simulink model "adcs_v16_integral_light_sun_sgp_igrf"  (Simulink 7.4)
settings: Solver=ode4  StartTime=0.0  StopTime=5000  FixedStep=s_SIM_STEP_SIZE  RelTol=1e-3
values from neighbouring files (symbols this model uses):
  A = ((T_SIDE + .29)*1e-3)^2    [constants_v13.m]    (also in constants_v15.m; constants_v15_Pow.m; constants_v15_Pow_ss_error.m; constants_v16_integral_kartavya.m)
  Bstar = SGP4dragp    (= -3.5889e-05)    [constants_v16_integral_light_sun_sgp_igrf_power_13Dec2011.m]    (also in getOrbitData.m = SGP4dragp; sgp.m = modTLE(4))
  Ca_Solar_Drag = 1.4    [constants_v13.m]    (also in constants_v15.m; constants_v15_Pow.m; constants_v15_Pow_ss_error.m; constants_v16_integral_kartavya.m)
  Cd = 2.2    [constants_v13.m]    (also in constants_v15.m; constants_v15_Pow.m; constants_v15_Pow_ss_error.m; constants_v16_integral_kartavya.m)
  check_time = 60000    [constants_v13.m]    (also in constants_v15.m = 10000; constants_v15_Pow.m = 10000; constants_v15_Pow_ss_error.m = 10000; constants_v16_integral_kartavya.m = 10000)
  ddn0 = 6*2*pi*SGPdragp2/(1440^3)    (= 0)    [constants_v16_integral_light_sun_sgp_igrf_power_13Dec2011.m]    (also in getOrbitData.m = 6*2*pi*SGPdragp2/(1440^3); sgp.m = modTLE(3))
  dn0 = 2*2*pi*SGPdragp1/(1440^2)    (= -4.7632944169e-11)    [constants_v16_integral_light_sun_sgp_igrf_power_13Dec2011.m]    (also in getOrbitData.m = 2*2*pi*SGPdragp1/(1440^2); sgp.m = modTLE(2))
  equinox = datenum('21-Mar-2010 12:0:0')    [constants_v13.m]    (also in constants_v15.m; constants_v15_Pow.m; constants_v15_Pow_ss_error.m; constants_v16_integral_kartavya.m)
  err_SGP = 0    [constants_v16_integral_kartavya.m]    (also in constants_v16_integral_light_sun_sgp_igrf_power_13Dec2011.m)
  i0 = pi*orbInc/180    (= 1.72229090587)    [constants_v16_integral_light_sun_sgp_igrf_power_13Dec2011.m]    (also in getOrbitData.m = pi*orbInc/180; sgp.m = modTLE(5))
  I_MAX = 0.5    [constants_v13.m]    (also in constants_v15.m; constants_v15_Pow.m; constants_v15_Pow_ss_error.m; constants_v16_integral_kartavya.m)
  I_TORQUER = 3.6 / 7.31    (= 0.492476060192)    [constants_v13.m]    (also in constants_v15.m; constants_v15_Pow.m; constants_v15_Pow_ss_error.m; constants_v16_integral_kartavya.m)
  Kd = 2* m_INERTIA / (s_numOrbits * T_ORBIT )    [constants_v13.m]    (also in constants_v15.m = m_INERTIA * (2 + delta)* zeta * w; constants_v15_Pow.m = m_INERTIA * (2 + delta)* zeta * w; constants_v15_Pow_ss_error.m = m_INERTIA * (2 + delta)* zeta * w; constants_v16_integral_kartavya.m = m_INERTIA * (2 + delta)* zeta * w)
  Kdetumb = K_det*eye(3)    [constants_v13.m]    (also in constants_v15.m; constants_v15_Pow.m; constants_v15_Pow_ss_error.m; constants_v16_integral_kartavya.m)
  Ki = m_INERTIA * delta * zeta * w^3    [constants_v15.m]    (also in constants_v15_Pow.m; constants_v15_Pow_ss_error.m; constants_v16_integral_kartavya.m; constants_v16_integral_light_sun_sgp_igrf_power_13Dec2011.m)
  Kp = m_INERTIA / (s_numOrbits * T_ORBIT * zeta)^2    [constants_v13.m]    (also in constants_v15.m = m_INERTIA * (w*w + 2*delta*zeta^2*w^2); constants_v15_Pow.m = m_INERTIA * (w*w + 2*delta*zeta^2*w^2); constants_v15_Pow_ss_error.m = m_INERTIA * (w*w + 2*delta*zeta^2*w^2); constants_v16_integral_kartavya.m = m_INERTIA * (w*w + 2*delta*zeta^2*w^2))
  M0 = pi*meanAno/180    (= 0)    [constants_v16_integral_light_sun_sgp_igrf_power_13Dec2011.m]    (also in getOrbitData.m = pi*meanAno/180; sgp.m = modTLE(9))
  m_INERTIA = [Ixx Ixy Ixz; Ixy Iyy Iyz; Ixz Iyz Izz]    [constants_v13.m]    (also in constants_v15.m; constants_v15_Pow.m = 1*[Ixx Ixy Ixz; Ixy Iyy Iyz; Ixz Iyz Izz]; constants_v15_Pow_ss_error.m = 1*[Ixx Ixy Ixz; Ixy Iyy Iyz; Ixz Iyz Izz]; constants_v16_integral_kartavya.m)
  mu = 6.673e-11*5.9742e24    (= 398658366000000)    [constants_v13.m]    (also in constants_v15.m; constants_v15_Pow.m; constants_v15_Pow_ss_error.m; constants_v16_integral_kartavya.m)
  N = 40    [constants_v13.m]    (also in constants_v15.m; constants_v15_Pow.m; constants_v15_Pow_ss_error.m; constants_v16_integral_kartavya.m)
  n0 = 2*pi*meanMo/1440    [constants_v16_integral_light_sun_sgp_igrf_power_13Dec2011.m]    (also in getOrbitData.m; sgp.m = modTLE(10))
  Ohm0 = pi*rghtAsc/180    (= 3.21433797681)    [constants_v16_integral_light_sun_sgp_igrf_power_13Dec2011.m]    (also in getOrbitData.m = pi*rghtAsc/180; sgp.m = modTLE(6))
  P_momentum_flux_from_the_sun = 4.4e-6    (= 4.4e-06)    [constants_v13.m]    (also in constants_v15.m; constants_v15_Pow.m; constants_v15_Pow_ss_error.m; constants_v16_integral_kartavya.m)
  q_BI0 = euler2qBI(roll0,pitch0,yaw0)    [constants_v13.m]    (also in constants_v15.m; constants_v15_Pow.m; constants_v15_Pow_ss_error.m; constants_v16_integral_kartavya.m)
  revNo = 1    [constants_v16_integral_kartavya.m]    (also in constants_v16_integral_light_sun_sgp_igrf_power_13Dec2011.m; precalcs.m; sgp.m = modTLE(11))
  s_AU = 159597870610    [constants_v16_integral_kartavya.m]    (also in constants_v16_integral_light_sun_sgp_igrf_power_13Dec2011.m; light_calc.m)
  s_FRAME_SIZE = 2    [constants_v13.m]    (also in constants_v15.m; constants_v15_Pow.m; constants_v15_Pow_ss_error.m; constants_v16_integral_kartavya.m)
  s_m_MAX = 0.95    [constants_v13.m]    (also in constants_v15.m; constants_v15_Pow.m; constants_v15_Pow_ss_error.m; constants_v16_integral_kartavya.m)
  s_MAG_B = 2.5e-5    (= 2.5e-05)    [constants_v13.m]    (also in constants_v15.m; constants_v15_Pow.m; constants_v15_Pow_ss_error.m; constants_v16_integral_kartavya.m)
  s_MAGMETER_WEIGHT = .9    (= 0.9)    [constants_v13.m]    (also in constants_v15.m; constants_v15_Pow.m; constants_v15_Pow_ss_error.m; constants_v16_integral_kartavya.m)
  s_Rearth = 6378164    [constants_v16_integral_kartavya.m]    (also in constants_v16_integral_light_sun_sgp_igrf_power_13Dec2011.m; light_calc.m)
  s_Rsun = 695500000    [constants_v16_integral_kartavya.m]    (also in constants_v16_integral_light_sun_sgp_igrf_power_13Dec2011.m; light_calc.m)
  s_SIM_STEP_SIZE = 0.1    [constants_v13.m]    (also in constants_v15.m; constants_v15_Pow.m; constants_v15_Pow_ss_error.m; constants_v16_integral_kartavya.m)
  s_SS_ADC_gain = 5    [constants_v13.m]    (also in constants_v15.m; constants_v15_Pow.m; constants_v15_Pow_ss_error.m; constants_v16_integral_kartavya.m)
  s_SS_ADC_res = 2^12 - 1    (= 4095)    [constants_v13.m]    (also in constants_v15.m; constants_v15_Pow.m; constants_v15_Pow_ss_error.m; constants_v16_integral_kartavya.m)
  s_SS_MAX_ANGLE = 85    [constants_v13.m]    (also in constants_v15.m; constants_v15_Pow.m; constants_v15_Pow_ss_error.m; constants_v16_integral_kartavya.m)
  s_TAU_W = 60    [constants_v13.m]    (also in constants_v15.m; constants_v15_Pow.m; constants_v15_Pow_ss_error.m; constants_v16_integral_kartavya.m)
  s_x_MAGMETER_BIAS = 50e-9    (= 5e-08)    [constants_v13.m]    (also in constants_v15.m; constants_v15_Pow.m; constants_v15_Pow_ss_error.m; constants_v16_integral_kartavya.m)
  s_YEAR = sime(1) + (sime(2)*30 - 30 + sime(3))/365    [constants_v16_integral_kartavya.m]    (also in constants_v16_integral_light_sun_sgp_igrf_power_13Dec2011.m; precalcs.m)
  side = 0.26    [constants_v13.m]    (also in constants_v15.m; constants_v15_Pow.m; constants_v15_Pow_ss_error.m; constants_v16_integral_kartavya.m)
  Snum = 6    [constants_v13.m]    (also in constants_v15.m; constants_v15_Pow.m; constants_v15_Pow_ss_error.m; constants_v16_integral_kartavya.m)
  t0 = (EpYear*meanYearDays + EpJD + EpTime)*1440    [constants_v16_integral_light_sun_sgp_igrf_power_13Dec2011.m]    (also in getOrbitData.m; sgp.m = modTLE(1))
  TLE_epoch = datenum('18-Oct-2010 10:30:0')    [constants_v16_integral_kartavya.m]    (also in constants_v16_integral_light_sun_sgp_igrf_power_13Dec2011.m; precalcs.m)
  today = datenum('18-Oct-2010 10:30:0')    [constants_v13.m]    (also in constants_v15.m; constants_v15_Pow.m; constants_v15_Pow_ss_error.m; constants_v16_integral_kartavya.m)
  tol_q4 = 0.7    [constants_v13.m]    (also in constants_v15.m = 0.85; constants_v15_Pow.m = 0.85; constants_v15_Pow_ss_error.m = 0.85; constants_v16_integral_kartavya.m = 0.85)
  tol_w = 4e-3    (= 0.004)    [constants_v13.m]    (also in constants_v15.m; constants_v15_Pow.m; constants_v15_Pow_ss_error.m; constants_v16_integral_kartavya.m)
  tolw_n2d = 10e-3    (= 0.01)    [constants_v15.m]    (also in constants_v15_Pow.m; constants_v15_Pow_ss_error.m; constants_v16_integral_kartavya.m; constants_v16_integral_light_sun_sgp_igrf_power_13Dec2011.m)
  Ts_display = 6    [constants_v13.m]    (also in constants_v15.m; constants_v15_Pow.m; constants_v15_Pow_ss_error.m; constants_v16_integral_kartavya.m)
  v_COM_to_COP_b = [.2; 1.75; .2]*1e-2    [constants_v13.m]    (also in constants_v15.m; constants_v15_Pow.m; constants_v15_Pow_ss_error.m; constants_v16_integral_kartavya.m)
  v_S1 = [1 0 0]    [constants_v13.m]    (also in constants_v15.m; constants_v15_Pow.m; constants_v15_Pow_ss_error.m; constants_v16_integral_kartavya.m)
  v_S2 = [-1 0 0]    [constants_v13.m]    (also in constants_v15.m; constants_v15_Pow.m; constants_v15_Pow_ss_error.m; constants_v16_integral_kartavya.m)
  v_S3 = [0 1 0]    [constants_v13.m]    (also in constants_v15.m; constants_v15_Pow.m; constants_v15_Pow_ss_error.m; constants_v16_integral_kartavya.m)
  v_S4 = [0 -1 0]    [constants_v13.m]    (also in constants_v15.m; constants_v15_Pow.m; constants_v15_Pow_ss_error.m; constants_v16_integral_kartavya.m)
  v_S5 = [0 0 1]    [constants_v13.m]    (also in constants_v15.m; constants_v15_Pow.m; constants_v15_Pow_ss_error.m; constants_v16_integral_kartavya.m)
  v_S6 = [0 0 -1]    [constants_v13.m]    (also in constants_v15.m; constants_v15_Pow.m; constants_v15_Pow_ss_error.m; constants_v16_integral_kartavya.m)
  v_x_MOUNTING_THETA_ZYX_BODY_TORQUER = [1; 1; 1]* pi/180    [constants_v13.m]    (also in constants_v15.m; constants_v15_Pow.m; constants_v15_Pow_ss_error.m; constants_v16_integral_kartavya.m)
  w0 = pi*argPer/180    (= 0)    [constants_v16_integral_light_sun_sgp_igrf_power_13Dec2011.m]    (also in getOrbitData.m = pi*argPer/180; sgp.m = modTLE(8))
  wx0 = 2*pi/180    (= 0.0349065850399)    [constants_v13.m]    (also in constants_v15.m = 0.00174532925199; constants_v15_Pow.m = 1.74532925199e-05; constants_v15_Pow_ss_error.m = 2.01533262693e-05; constants_v16_integral_kartavya.m = 0.0174532925199)
  wy0 = 1*pi/180    (= 0.0174532925199)    [constants_v13.m]    (also in constants_v15.m = 0.00174532925199; constants_v15_Pow.m = 1.74532925199e-05; constants_v15_Pow_ss_error.m = 2.01533262693e-05; constants_v16_integral_kartavya.m = 0)
  wz0 = -2*pi/180    (= -0.0349065850399)    [constants_v13.m]    (also in constants_v15.m = 0.00174532925199; constants_v15_Pow.m = 1.74532925199e-05; constants_v15_Pow_ss_error.m = 2.01533262693e-05; constants_v16_integral_kartavya.m = -0.00872664625997)
undefined symbols (not defined in the file or in its folder): agh, agh41, dgh, dgh41
libraries: commnoisgen2 x7, simulink x4, aerolibutil x2, dspmtrx3 x1
(part 2 of 2)

== matlab function External Torques/Subsystem/Solar_drag ==
  data: v_Sun_b input double; solar_drag output double; Ca_Solar_Drag parameter double; P_momentum_flux_from_the_sun parameter double; light input double; side parameter double
function solar_drag = fcn(v_Sun_b,Ca_Solar_Drag,P_momentum_flux_from_the_sun,light, side)
% This block supports the Embedded MATLAB subset.
% See the help menu for details. 

% dot product of area vector and sun vector
if (norm(v_Sun_b) == 0)
    u = [1;0;0];
else
    u = v_Sun_b / norm(v_Sun_b);
end

y = 0 ;
a = side;
a = a*a; %Area of satellite
b =  zeros(3,6);
b(:,1) = a*[1;0;0];
b(:,2) = a*[0;1;0];
b(:,3) = a*[0;0;1];
b(:,4) = a*[-1;0;0];
b(:,5) = a*[0;-1;0];
b(:,6) = a*[0;0;-1];

x = 0;
for i=1:6
     x = dot(b(:,i),u);
    if(x>0)
            y = y+x;
    end
end
Ap = y;

solar_drag = -Ap * Ca_Solar_Drag * P_momentum_flux_from_the_sun * u * light;

== matlab function External Torques/L_Inertial ==
  data: x input double; tau output double; v_Si input double; mu parameter double; m_INERTIA parameter double
function tau = fcn(x, v_Si, mu, m_INERTIA)
% This block supports the Embedded MATLAB subset.
% See the help menu for details. 

q = x(1:4);

q0 = q(4); q1 = q(1); q2 = q(2); q3 = q(3);

TBI = [ q0^2 + q1^2 - q2^2 - q3^2,         2*q0*q3 + 2*q1*q2,         2*q1*q3 - 2*q0*q2;
           2*q1*q2 - 2*q0*q3, q0^2 - q1^2 + q2^2 - q3^2,         2*q0*q1 + 2*q2*q3;
           2*q0*q2 + 2*q1*q3,         2*q2*q3 - 2*q0*q1, q0^2 - q1^2 - q2^2 + q3^2];

r_I = v_Si(1:3);
r_B =  TBI*r_I;

R = sqrt(dot(r_B, r_B));
tau = 3*mu * cross( r_B, m_INERTIA*r_B) / R^5;

== matlab function Control Law/q->w ==
  data: B output double; B_l input double; B_k input double; dB output double; s_FRAME_SIZE parameter double
function [B, dB] = fcn(B_l, B_k, s_FRAME_SIZE)
% This block supports the Embedded MATLAB subset.
% See the help menu for details. 

dB = (B_l - B_k)/s_FRAME_SIZE;
B = (B_l + B_k)/2;

== matlab function QuEST ==
  data: v_Bb_m input double; m_SUN input double; q_BO_est output double; v_Bo_c input double; v_So_c input double; s_SS_ADC_gain parameter double; Snum parameter double; light_est output double; s_MAGMETER_WEIGHT parameter double; s_SS_MAX_ANGLE parameter double; v_Sun1 output double
function [q_BO_est, light_est, v_Sun1] = QuEST(v_Bb_m,m_SUN,v_Bo_c,v_So_c, s_SS_ADC_gain, Snum, s_MAGMETER_WEIGHT, s_SS_MAX_ANGLE)

    % Help
    % q_triad = Estimated quaternion
    % b1,b2 = the 2 measurement vectors in body frames
    % r1,r2 = the 2 measurement vectors in reference frames (orbit/inertial; orbit used)
    % b1 is the measurement with very high accurace as compared to b2
    % I am not sure how r1 and r2 will be determined
    % a1 and a2 are Relative weights of b1 and b2


%%%%% calculate v_Sb_m from m_SUN %%%%
t_S = ones(1,Snum)*cos(s_SS_MAX_ANGLE *pi/180);
m_SUN(4,:) = 1.0*(m_SUN(5,:)>t_S);     % set flags from measured voltages

values = m_SUN(5,:);

n_SS = 0;
for i=1:Snum
    if values(i) < 0.5*s_SS_ADC_gain
        n_SS = n_SS + 1;
    end
end

if (n_SS == Snum) 
    light = 0;
else
    light = 1;
end

light_est = light;
%v_Sun1 = [1;0;0];

if (light == 1)    
    
    %%% CALCULATE SUN VECTOR %%%
    
    ssvectors = zeros(3); ssvalues = zeros(3,1); ssflags = zeros(3,1);
     % flags = m_SUN(4,:)';
%     for i=1:3
%         [~, index] = sort(m_SUN(5,:));  % sort values in ascending order
%         z = index(Snum);
%         ssvectors(i,1:3) = m_SUN(1:3,z)';
%         ssflags(i) = m_SUN(4,z);
%         ssvalues(i) = m_SUN(5,z);
%         m_SUN(5,z) = -100 ;
%         for j= 1:Snum
%             if( norm(ssvectors(i,1:3)+m_SUN(1:3,j)') == 0 )
%                 m_SUN(5,j) = -100;
%             end
%         end
%     end
    
    [~, index] = sort(m_SUN(5,:));  % sort values in ascending order
    z = index(Snum); p = 0; % first vector
    ssvectors(1,1:3) = m_SUN(1:3,z)';
    ssvalues(1) = m_SUN(5,z);
    p = p+1;
    
    z = index(Snum-p);  % second vector
    while norm(m_SUN(1:3,z)' + ssvectors(1,1:3)) == 0
        p = p+1;
        z = index(Snum - p);
    end
    ssvectors(2,1:3) = m_SUN(1:3,z)';
    ssvalues(2) = m_SUN(5,z);
    p = p+1;
    
    z = index(Snum-p);  % 3rd vector
    while (norm(m_SUN(1:3,z)' + ssvectors(1,1:3)) == 0) || (norm(m_SUN(1:3,z)' + ssvectors(2,1:3)) == 0)
        p = p+1;
        z = index(Snum - p);
    end
    ssvectors(3,1:3) = m_SUN(1:3,z)';
    ssvalues(3) = m_SUN(5,z);
%     p = p+1;
    
    % v_Sun1 = inv(ssvectors)*ssvalues;
    v_Sun1 = ssvectors\ssvalues;
    v_Sun1 = v_Sun1/sqrt(dot(v_Sun1, v_Sun1));
    v_Sb_m = v_Sun1/sqrt(dot(v_Sun1, v_Sun1));
    
    %%%% start TRIAD %%%%

    b1 = v_Bb_m;
    b2 = v_Sb_m;
    r1 = v_Bo_c;
    r2 = v_So_c;

    a1 = s_MAGMETER_WEIGHT;
    a2 = 1-a1;

    %b3
    b3 = cross(b1,b2);
    b3 = b3/norm(b3) ;
    %r3
    r3 = cross(r1,r2);
    r3 = r3/norm(r3) ;

    %mu
    mu = ( 1 + dot(b3,r3) ) * ( a1*dot(b1,r1) + a2*dot(b2,r2) ) ;
    mu =  mu + dot( cross(b3,r3) , ( a1*cross(b1,r1) + a2*cross(b2,r2) ) ) ;

    %nu
    nu = dot( ( b3 + r3 ) , ( a1*cross(b1,r1) + a2*cross(b2,r2) )  ) ;

    %rho
    rho = sqrt( mu*mu + nu*nu );

    %q
    if( mu > 0)
        k_q_triad = (1/( 2*sqrt( rho*(rho+mu)*( 1 + dot(b3,r3) ) ) ) );
        v_q_triad = ( rho + mu )*( cross(b3,r3) ) + nu*(b3 + r3) ;
        s_q_triad = ( rho + mu )* ( 1 + dot(b3,r3) ) ;
        q_triad = [v_q_triad ; s_q_triad];
        q_triad = k_q_triad * q_triad ;
    else
        k_q_triad = (1/( 2*sqrt( rho*(rho-mu)*( 1 + dot(b3,r3) ) ) ) );
        v_q_triad = ( nu )*( cross(b3,r3) ) + ( rho - mu )*(b3 + r3) ;
        s_q_triad = ( nu )* ( 1 + dot(b3,r3) ) ;
        q_triad = [v_q_triad ; s_q_triad];
        q_triad = k_q_triad * q_triad ;    
    end

    q_triad = q_triad / sqrt(dot(q_triad,q_triad)) ;
    q_BO_est = q_triad;
else
    v_Sun1 = [1 ; 0 ; 0];
    q_BO_est = [0;0;0;1];
    flag_sum = 0;
end
end

== matlab function Satellite Computations I Propagators/m_TOI_NEW1 ==
  data: v_I input double; ECI input double; v_O output double
function v_O  = fcn(v_I, ECI)
% This block gives DCM for converting from ECI to ORBIT frames
% inputs: state vector in ECI
% output: DCM

r = ECI(1:3);   % position vector in ECI
v = ECI(4:6);   % velocity vector in ECI

oy = cross(v,r);    % orbit frame x...
oy = oy/sqrt(dot(oy,oy));

oz = -r/sqrt(dot(r,r));

ox = cross(oy,oz);
ox = ox/sqrt(dot(ox,ox));

TOI = [ox oy oz]';

v_O = TOI*v_I;

== matlab function Control Law/Nominal ==
  data: ieu output double; ieu_prev input double; eu output double; m output double; light input double; w input double; m_N output double; v_B input double; Kp parameter double; Kd parameter double; Ki parameter double; q input double; s_FRAME_SIZE parameter double
function [ieu, eu, m, m_N] = fcn(ieu_prev, light, w, v_B, Kp, Kd, Ki, q, s_FRAME_SIZE)
% This block supports the Embedded MATLAB subset.
% See the help menu for details. 

Bnorm = sqrt(dot(v_B, v_B));

q = q/sqrt(dot(q,q));

qv = q(1:3);    % e*sin(t/2)
qs = q(4);      %   cos(t/2)

eu = 2*qv*qs;     % 2*e*sin(t/2)*cos(t/2) = e*sin(t)    % P variable
         
ieu = ieu_prev + eu*s_FRAME_SIZE;   % integral eu dt,   % I variable

m = (Kp*eu + Ki*ieu + Kd*w) / Bnorm^2;

m_N = cross( m, v_B ) * light;

== matlab function IGRF /ECI -> LLA/r_ECEF -> r_LLA ==
  data: r_ECEF input double; Latitude output double; Longitude output double; Altitude output double
function [Latitude, Longitude, Altitude] = fcn(r_ECEF)
%r_ECEF: ECEF position vector (in m)
%r_LLA: LLA postion vector (in rad, m)

% CHATI
% radius_earth = 6371000;
% r = norm(r_ECEF);
% x = r_ECEF(1);
% y = r_ECEF(2);
% z = r_ECEF(3);
% 
% lat = asin(z/r);
% long = atan2(y,x);
% if (long < 0)
%     long = long + 2*pi;
% end
% h = r - radius_earth;
% 
% Latitude = lat*180/pi; %deg
% Longitude = long*180/pi; %deg
% Altitude  = h/1000; %km
%r_LLA = [lat;long;h];

% 
% MATLAB
% L = ecef2lla(r_ECEF);
% Latitude = L(1); % deg
% Longitude = L(2); % deg
% Altitude = L(3)/1000; % km


% JAIDEEP
x = r_ECEF(1);
y = r_ECEF(2);
z = r_ECEF(3);

% wgs84model
f  = 1/298.257223563; % flattening
R =  6378137; % equatorial radius

% [phi, lambda, h] = ecef2geodetic(p(:,1), p(:,2), p(:,3), [R sqrt( 1 - ( 1 - f )^2 )]);
% Ellipsoid constants
% ellipsoid = [R sqrt( 1 - ( 1 - f )^2 )];
a  = R; % ellipsoid(1);       % Semimajor axis
e2 =  1 - ( 1 - f )^2; % ellipsoid(2) ^ 2;   % Square of first eccentricity
ep2 = e2 / (1 - e2);     % Square of second eccentricity
% f = 1 - sqrt(1 - e2);    % Flattening
b = a * (1 - f);         % Semiminor axis

% Longitude
lambda = atan2(y,x);

% Distance from Z-axis
rho = sqrt(x^2 + y^2);

% Bowring's formula for initial parametric (beta) and geodetic (phi) latitudes
beta = atan2(z, (1 - f) * rho);
phi = atan2(z   + b * ep2 * sin(beta).^3,...
            rho - a * e2  * cos(beta).^3);

% Fixed-point iteration with Bowring's formula
% (typically converges within two or three iterations)
betaNew = atan2((1 - f)*sin(phi), cos(phi));
count = 0;
while any(beta(:) ~= betaNew(:)) && count < 5
    beta = betaNew;
    phi = atan2(z   + b * ep2 * sin(beta).^3,...
                rho - a * e2  * cos(beta).^3);
    betaNew = atan2((1 - f)*sin(phi), cos(phi));
    count = count + 1;
end

% Calculate ellipsoidal height from the final value for latitude
sinphi = sin(phi);
N = a ./ sqrt(1 - e2 * sinphi.^2);
h = rho .* cos(phi) + (z + e2 * N .* sinphi) .* sinphi - N;

Latitude = phi*180/pi;
Longitude = lambda*180/pi;
Altitude = h/1000;  % km

== matlab function IGRF /ECI -> LLA/r_ECI -> r_ECEF ==
  data: today parameter double; r_ECEF output double; equinox parameter double; v_S_i input double; t input double
function r_ECEF = fcn(today,equinox,v_S_i,t)
%u: position vector in ECI (in m)
%y: position vector in ECEF (in m)

r_I = v_S_i(1:3);

stperut = 1.00273790935;    % siderial time = stperut * universal time
W_EARTH_ROT = 2*pi/86141;   % sidereal rotation angular velocity of earth, SI

ut_sec = (today - equinox)*24*60*60 + t; % universal time vector in sec
st_sec = stperut*ut_sec;    % sidereal time vector in sec

phi = st_sec*W_EARTH_ROT;            % sidereal time vector in rad

TEI = [ cos(phi) sin(phi) 0;
       -sin(phi) cos(phi) 0;
        0        0        1];

r_ECEF = TEI*r_I;

== matlab function External Torques/Aerodynamic Torque/aero torque ==
  data: rho input double; v_B input double; u_aero output double; side parameter double; Cd parameter double; v_COM_to_COP_b parameter double
function u_aero = fcn(rho, v_B,side, Cd, v_COM_to_COP_b)

% x = 1;
% z = x*1;
% y = z*u;

% This block supports an embeddable subset of the MATLAB language.
% See the help menu for details. 
% dot product of area vector and velocity vector

vnorm = sqrt(dot(v_B,v_B));
v_unit = v_B / vnorm;

y = 0 ;
a = side;
a = a*a; %Area of satellite
b =  zeros(3,6);
b(:,1) = a*[1;0;0];
b(:,2) = a*[0;1;0];
b(:,3) = a*[0;0;1];
b(:,4) = a*[-1;0;0];
b(:,5) = a*[0;-1;0];
b(:,6) = a*[0;0;-1];

for i=1:6
     x = dot(b(:,i),v_unit);
    if(x>0)
            y = y+x;
    end
end
Ap = y; % total exposed area

F_aero = -0.5 * Cd * rho * Ap * vnorm^2 * v_unit;

u_aero = cross(v_COM_to_COP_b, F_aero);

== matlab function IGRF /Embedded MATLAB Function ==
  data: ALT input double; Bi output double; LAT input double; ELONG input double; DATE input double; ORDER input double; agh parameter double; agh41 parameter double; dgh parameter double; dgh41 parameter double
function  Bi = igrf1(ALT,LAT,ELONG,DATE, ORDER, agh, agh41, dgh, dgh41)
%  MAGFD
%  Function to compute Earths magnetic field
%  and components: X,Y,Z,T for a given latitude
%  and longitude, date and altitude.
%  Uses MATLAB MAT files sh1900.mat to sh2010.mat in 5 yr
%  intervals. ONLY uses harmonic expansion to order 10 at present.
%
%  Usage: out=magfd(DATE,ITYPE,ALT,COLAT,ELONG);
%
%  DATE = date of survey (decimal years)
%  ITYPE=1 for geodetic coordinates (usual case)
%  ITYPE=2 for geocentric coordinates
%  ALT = (for ITYPE=1) altitude of survey relative to sealevel (km +ve up)
%  ALT = (for ITYPE=2) radial distance from center of earth in km
%  COLAT=90-latitude (decimal degrees)
%  ELONG=longitude of survey (decimal degrees)
%
%  Output array out contains components X,Y,Z,T in nanoteslas
%   X north component
%   Y east component     
%   Z vertical component +ve down
%   T total field magnitude
%
%  ref: IAGA, Division V, Working Group VMOD, 
%   The 10th generation International Geomagnetic 
%   Reference Field, Geophys. J. Int, 161, 561-565, 2005.
%
% Maurice A. Tivey March 1997
% Mod Dec 1999 (add igrf2000 and y2k compliance
% Mod Nov 2000 (use up to degree 10 sh coefficients)
% Mod Apr 2005 added 2005 coeffs
% Mod Sep 2006 some clean up and info added
% Mod Jan 2010 added 2010 coefficients
% http://deeptow.whoi.edu/matlab.html
% Copyright: Maurice A. Tivey, 2005
%  Woods Hole Oceanographic Institution

ITYPE = 1;
COLAT = 90- LAT;
CL = zeros(1,14);
SL = zeros(1,14);
P = zeros(1,104);
Q = zeros(1,104);
RR = 0;
FN = 0;

DGRF= 1000:5:2010;
igrfyear=2010;
% igrffile='sh2010';
% 
% pl=0;
% if DATE < 0, pl=1; end
% DATE=abs(DATE);
% Determine year for base DGRF to use.
% if DATE < igrfyear,
%     T =0;
%       BASE=fix(DATE-DGRF(1)); 
%       i=fix(BASE/5)+1;
%       BASE=DGRF(i);
% %       if pl==0,
% %           fprintf('Using DGRF base year %f \n',BASE);      
% %       end
%       eval(['load sh',num2str(BASE)])
%       % loads agh and agh41 but now need to get next epoch
%        iagh=agh;iagh41=agh41;
%       % figure out next epoch to load
%       if BASE < 1900, % a check to get pre-1900 estimates of gauss coeffs
%        eval(['load sh',num2str(BASE+25)])
%       else
%        eval(['load sh',num2str(DGRF(i+1))])
%       end
%        eagh=agh;eagh41=agh41;
%        dgh=(eagh-iagh)./5;dgh41=(eagh41-iagh41)./5;
%        agh=iagh;agh41=iagh41;
%        clear iagh iagh41 eagh eagh41
%        T = DATE - BASE;
% else
%       if pl==0,
%           fprintf('Using IGRF base year %f \n',igrfyear);       
%       end
%       eval(['load ',igrffile])   % load in igrf data file
      T     = DATE - igrfyear;
% end
% combine spherical harmonic coefficients from first 8 degrees 
% with degrees 9 thru 13 

 agh_full=[agh,agh41];
 dgh_full=[dgh,dgh41];
%
      D2R   = pi/180;
      R     = ALT;
      SLAT  = cos(COLAT*D2R);
      CLAT  = sin(COLAT*D2R);
      CL(1) = cos(ELONG*D2R);
      SL(1) = sin(ELONG*D2R);
      X     = 0.0;
      Y     = 0.0;
      Z     = 0.0;
      CD    = 1.0;
      SD    = 0.0;
      L     = 1;
      M     = 1;
      N     = 0;
      RE    = 6371.2; % Earth's mean radius
if ITYPE == 1  % CONVERSION FROM GEODETIC TO GEOCENTRIC COORDINATES
	%A2    = 40680925.;  % squared semi major axis
	%B2    = 40408588.;  % squared semi minor axis
    % WGS84
	A2    = 40680631.59; % 6378.137^2; % squared semi major axis
	B2    = 40408299.98; % 6356.7523142^2; % squared semi minor axis
	ONE   = A2*CLAT*CLAT;
	TWO   = B2*SLAT*SLAT;
	THREE = ONE + TWO;
	FOUR  = sqrt(THREE);
	R     = sqrt(ALT*(ALT + 2.0*FOUR) + (A2*ONE + B2*TWO)/THREE);
	CD    = (ALT + FOUR)/R;
	SD    = (A2 - B2)/FOUR*SLAT*CLAT/R;
	ONE   = SLAT;
	SLAT  = SLAT*CD - CLAT*SD;
	CLAT  = CLAT*CD +  ONE*SD;
end
% if geocentric coordinates desired then only need to define the following
	RATIO = RE/R;
%
%     COMPUTATION OF SCHMIDT QUASI-NORMAL COEFFICIENTS  P AND X(=Q)
%
      P(1)  = 2.0*SLAT;
      P(2)  = 2.0*CLAT;
      P(3)  = 4.5*SLAT*SLAT - 1.5;
      P(4)  = sqrt(27)*CLAT*SLAT;
      Q(1)  = -CLAT;
      Q(2)  =  SLAT;
      Q(3)  = -3.0*CLAT*SLAT;
      Q(4)  = sqrt(3)*(SLAT*SLAT - CLAT*CLAT);

NMAX=ORDER; % Max number of harmonic degrees
NPQ=(NMAX*(NMAX+3))/2;
for K=1:NPQ,
 if N < M 
	M     = 0;
	N     = N + 1;
	RR    = RATIO^(N + 2);
	FN    = N;
 end
 FM    = M;
 if K >= 5 %8,5,5
	if (M-N) == 0 %,7,6,7
		ONE   = sqrt(1.0 - 0.5/FM);
		J     = K - N - 1;
		P(K)  = (1.0 + 1.0/FM)*ONE*CLAT*P(J);
		Q(K)  = ONE*(CLAT*Q(J) + SLAT/FM*P(J));
		SL(M) = SL(M-1)*CL(1) + CL(M-1)*SL(1);
		CL(M) = CL(M-1)*CL(1) - SL(M-1)*SL(1);
	else
		ONE   = sqrt(FN*FN - FM*FM);
		TWO   = sqrt((FN - 1.0)^2 - FM*FM)/ONE;
		THREE = (2.0*FN - 1.0)/ONE;
		I     = K - N;
		J     = K - 2*N + 1;
		P(K)  = (FN + 1.0)*(THREE*SLAT/FN*P(I) - TWO/(FN - 1.0)*P(J));
		Q(K)  = THREE*(SLAT*Q(I) - CLAT/FN*P(I)) - TWO*Q(J);
	end
%
%     SYNTHESIS OF X, Y AND Z IN GEOCENTRIC COORDINATES
%
 end
 ONE   = (agh_full(L) + dgh_full(L)*T)*RR;

 if M == 0 %10,9,10
	X     = X + ONE*Q(K);
	Z     = Z - ONE*P(K);
	L     = L + 1;
 else
	TWO   = (agh_full(L+1) + dgh_full(L+1)*T)*RR;
	THREE = ONE*CL(M) + TWO*SL(M);
	X     = X + THREE*Q(K);
	Z     = Z - THREE*P(K);
	if CLAT > 0 %12,12,11
		Y = Y+(ONE*SL(M)-TWO*CL(M))*FM*P(K)/((FN + 1.0)*CLAT);
	else
		Y = Y + (ONE*SL(M) - TWO*CL(M))*Q(K)*SLAT;
	end
	L     = L + 2;
 end
	M     = M + 1;
end
%     CONVERSION TO COORDINATE SYSTEM SPECIFIED BY ITYPE

ONE   = X;
X     = X*CD +  Z*SD;
Z     = Z*CD - ONE*SD;
T     = sqrt(X*X + Y*Y + Z*Z);
Bi=[X,Y,Z];
%  END

== matlab function IGRF /Embedded MATLAB Function1 ==
  data: B_I output double; LAT input double; LONG input double; B_NED input double; today parameter double; equinox parameter double; t input double
function B_I = fcn(LAT, LONG, B_NED, today, equinox, t)
%#eml

stperut = 1.00273790935;    % siderial time = stperut * universal time
W_EARTH_ROT = 2*pi/86141;   % sidereal rotation angular velocity of earth, SI

ut_sec = (today - equinox)*24*60*60 + t; % universal time vector in sec
st_sec = stperut*ut_sec;    % sidereal time vector in sec

phi = st_sec*W_EARTH_ROT;            % sidereal time vector in rad

TEI = [ cos(phi) sin(phi) 0;
       -sin(phi) cos(phi) 0;
        0        0        1];


    
angles = [LAT LONG]*pi/180;

dcm = zeros(3,3,size(angles,1));  % dcmeceeftoned    
cang = cos( angles );
sang = sin( angles );

dcm(1,1,:) = -cang(:,2).*sang(:,1);
dcm(1,2,:) = -sang(:,2).*sang(:,1);
dcm(1,3,:) = cang(:,1);
dcm(2,1,:) = -sang(:,2);
dcm(2,2,:) = cang(:,2);
dcm(2,3,:) = 0.0;
dcm(3,1,:) = -cang(:,2).*cang(:,1);
dcm(3,2,:) = -sang(:,2).*cang(:,1);
dcm(3,3,:) = -sang(:,1);

B_ECEF = dcm'*B_NED';

B_I = TEI'*B_ECEF;

== matlab function External Torques/Aerodynamic Torque/v_I to v_B ==
  data: v_I input double; x input double; v_B output double
function v_B = fcn(v_I,x)
% This block supports the Embedded MATLAB subset.
% See the help menu for details. 

q = x(1:4);

q0 = q(4); q1 = q(1); q2 = q(2); q3 = q(3);

TBI = [ q0^2 + q1^2 - q2^2 - q3^2,         2*q0*q3 + 2*q1*q2,         2*q1*q3 - 2*q0*q2;
           2*q1*q2 - 2*q0*q3, q0^2 - q1^2 + q2^2 - q3^2,         2*q0*q1 + 2*q2*q3;
           2*q0*q2 + 2*q1*q3,         2*q2*q3 - 2*q0*q1, q0^2 - q1^2 - q2^2 + q3^2];

v_B =  TBI*v_I;

== matlab function Eclipse model/Eclipse Model ==
  data: s_AU input double; flag output double; s_Rearth input double; s_Rsun input double; v_S_i input double; v_Sun_i input double; alpha output double; beta output double; parameter_umbra output double; parameter_penumbra output double
function [flag, alpha, beta, parameter_umbra, parameter_penumbra] = fcn(s_AU, s_Rearth, s_Rsun, v_S_i, v_Sun_i)
% This block supports the Embedded MATLAB subset.
% See the help menu for details. 

%159597870610 m = 1 AU
%695500000 m = Sun radius

v_pos_S_i = v_S_i(1:3);

% umbra = s_AU*s_Rearth / (s_Rsun - s_Rearth);
% penumbra = s_AU*s_Rearth / (s_Rsun + s_Rearth);
% 
% alpha = asin(s_Rearth / umbra);
% beta = asin(s_Rearth / penumbra);
% 
% angle_sat = acos(dot(v_pos_S_i, v_Sun_i) / norm(v_pos_S_i));
% 
% parameter_umbra = acos((dot((v_pos_S_i + umbra*v_Sun_i), v_Sun_i)) / norm(v_pos_S_i + umbra*v_Sun_i));
% parameter_penumbra = acos((dot((v_pos_S_i - penumbra*v_Sun_i), -v_Sun_i)) / norm(v_pos_S_i - penumbra*v_Sun_i));
% 
% flag = 1;
% 
% if ((angle_sat >= pi/2 + alpha) && (parameter_umbra <= alpha))
%     flag = 0;
% elseif ((angle_sat >= pi/2 + beta) && (parameter_umbra > alpha) && (parameter_penumbra <= beta))
%         flag = 0.5;
% end

%% this code take from light_calc.m
    umbra = s_AU*s_Rearth / (s_Rsun - s_Rearth);
    penumbra = s_AU*s_Rearth / (s_Rsun + s_Rearth);

    alpha = asin(s_Rearth / umbra);
    beta = asin(s_Rearth / penumbra);

    angle_sat = acos(dot(v_pos_S_i, v_Sun_i) / norm(v_pos_S_i));

    parameter_umbra = acos((dot((v_pos_S_i + umbra*v_Sun_i), v_Sun_i)) / norm(v_pos_S_i + umbra*v_Sun_i));
    parameter_penumbra = acos((dot((v_pos_S_i - penumbra*v_Sun_i), -v_Sun_i)) / norm(v_pos_S_i - penumbra*v_Sun_i));

    flag = 1;

    if ((angle_sat >= pi/2 + alpha) && (parameter_umbra <= alpha))
        flag = 0;
    elseif ((angle_sat >= pi/2 + beta) && (parameter_umbra > alpha) && (parameter_penumbra <= beta))
        flag = 0.5;
    end

== matlab function Sensors1/Sun Sensors/Embedded MATLAB Function ==
  data: v_S1 input double; m_SUN output double; s_S1 input double; v_S2 input double; s_S2 input double; v_S3 input double; s_S3 input double; v_S4 input double; s_S4 input double; v_S5 input double; s_S5 input double; v_S6 input double; s_S6 input double; Snum parameter double; s_SS_MAX_ANGLE parameter double; values output double
function [m_SUN, values] = fcn(v_S1, s_S1, v_S2, s_S2, v_S3, s_S3, v_S4, s_S4, v_S5, s_S5, v_S6, s_S6, Snum, s_SS_MAX_ANGLE)

a = cos(s_SS_MAX_ANGLE *pi/180);
t_S = ones(1,6)*a;

m_SUNtot = [v_S1 v_S2 v_S3 v_S4 v_S5 v_S6 ; % SS vectors
               0    0    0    0    0    0 ; % flags
            s_S1 s_S2 s_S3 s_S4 s_S5 s_S6 ];% values
        
m_SUNtot(4,:) = 1.0*(m_SUNtot(5,:)>t_S);

m_SUN = m_SUNtot(:, 1:Snum);
values = m_SUN(5,:)';

== matlab function Control Law/Detumbling ==
  data: v_B input double; Bdot input double; Kdetumb parameter double; m_D output double; s_MAG_B parameter double
function m_D = fcn(v_B, Bdot, Kdetumb, s_MAG_B)
% This block supports the Embedded MATLAB subset.
% See the help menu for details. 

Bnorm = sqrt(dot(v_B, v_B));
m_D = -Kdetumb * Bdot * (s_MAG_B / Bnorm);

== matlab function Control Law/Switching Algorithm/gate pulse ==
  data: N_prev input double; w input double; q input double; tol_w parameter double; tolw_n2d parameter double; N output double; P output double; tol_q4 parameter double; t input double; check_time parameter double; light_flag input double; w_ctrl input double; t_now output double; t_now_prev input double
function [N,P,t_now] = fcn( N_prev, w, q, tol_w, tolw_n2d, tol_q4, t,check_time, light_flag, w_ctrl,t_now_prev)

modw = sqrt(dot(w, w));
switch_d2n = (modw < tol_w) && (light_flag*w_ctrl ==1);
switch_n2d = (modw > tolw_n2d);

% condition check - DEBUG purpose
P = [1.0*(abs(q(4)) > tol_q4) + 0.1; 
     1.0*(modw < tol_w);
     1.0*(light_flag*w_ctrl == 1) + 0.3];
%%%%%%%%%%%

N = N_prev;
t_now = t_now_prev;

if t < 2000
    N = 0;
    t_now = 0;
end

if ((switch_d2n == 1) && (N_prev == 0))
    N = 1;
    t_now = t;
end

if ((switch_n2d == 1) && (N_prev == 1) && (t > t_now_prev + check_time) )
    N = 0;
    t_now = t;
end

== matlab function Satellite Computations I Propagators/m_TOI_NEW ==
  data: ECI input double; v_O output double; v_I input double
function v_O  = fcn(ECI, v_I)
% This block gives DCM for converting from ECI to ORBIT frames
% inputs: state vector in ECI
% output: DCM

r = ECI(1:3);   % position vector in ECI
v = ECI(4:6);   % velocity vector in ECI

oy = cross(v,r);    % orbit frame x...
oy = oy/sqrt(dot(oy,oy));

oz = -r/sqrt(dot(r,r));

ox = cross(oy,oz);
ox = ox/sqrt(dot(ox,ox));

TOI = [ox oy oz]';

v_O = TOI*v_I;

== matlab function q -> w/q->w ==
  data: w_l output double; w_k input double; q_BI_l input double; q_BI_k input double; w output double; s_FRAME_SIZE parameter double; s_TAU_W parameter double
function [w_l,w] = fcn(w_k, q_BI_l, q_BI_k, s_FRAME_SIZE, s_TAU_W)
% This block supports the Embedded MATLAB subset.
% See the help menu for details. 
dq = (q_BI_l - q_BI_k)/s_FRAME_SIZE;
q = (q_BI_l + q_BI_k)/2;

de = dq(1:3);
e = q(1:3);
n = q(4);

ex = [0    -e(3)  e(2);
      e(3)     0 -e(1);
     -e(2)  e(1)    0];

w = 2*(n*n*eye(3) - n*ex + e*e')*de/n;

% filtering:

a = s_FRAME_SIZE/(s_FRAME_SIZE + s_TAU_W);
w_l = a*w + (1-a)*w_k;

== matlab function Embedded MATLAB Function4 ==
  data: x input double; euler output double; v_Si input double; q_BO output double; w_BOB output double; modw output double; s_W_SAT parameter double; w_BIB output double
function [euler, q_BO, w_BOB, modw, w_BIB] = a(x,v_Si, s_W_SAT)
% This block supports the Embedded MATLAB subset.
% See the help menu for details. 

% ECI to TIO 
r = v_Si(1:3);   % position vector in ECI
v = v_Si(4:6);   % velocity vector in ECI

oy = cross(v,r);    % orbit frame x...
oy = oy/sqrt(dot(oy,oy));

oz = -r/sqrt(dot(r,r));

ox = cross(oy,oz);
ox = ox/sqrt(dot(ox,ox));

TIO = [ox oy oz];

% qIO from TIO
if (trace(TIO) == -1)
    if ( TIO(1,2) == 0 && TIO(1,3) ==0 )
        q_IO = [1; 0; 0; 0];
    elseif ( TIO(1,2) == 0 && TIO(2,3) ==0 )
        q_IO = [0; 1; 0; 0];
    elseif ( TIO(1,3) == 0 && TIO(2,3) ==0 )
        q_IO = [0; 0; 1; 0];
    else
        e1 = TIO(1,2)*TIO(1,3);
        e2 = TIO(1,2)*TIO(2,3);
        e3 = TIO(1,3)*TIO(2,3);
        norm = sqrt( e1*e1 + e2*e2 + e3*e3);
        q_IO = [e1; e2; e3; 0]/norm;
    end        
else
    q4 = 0.5*sqrt(1 + trace(TIO));
    q1 = -(TIO(3,2) - TIO(2,3)) / (4*q4);
    q2 = -(TIO(1,3) - TIO(3,1)) / (4*q4);
    q3 = -(TIO(2,1) - TIO(1,2)) / (4*q4);
    q_IO = [q1; q2; q3; q4];
end

q_BI = x(1:4);

% q_BO = q_BI*q_IO
q_BIx = ...
[ q_BI(4)  q_BI(3) -q_BI(2) q_BI(1);
 -q_BI(3)  q_BI(4)  q_BI(1) q_BI(2);
  q_BI(2) -q_BI(1)  q_BI(4) q_BI(3);
 -q_BI(1) -q_BI(2) -q_BI(3) q_BI(4)];

q_BO = q_BIx * q_IO;

euler =  (180/pi)*[atan2( 2*( q_BO(4)*q_BO(1)-q_BO(2)*q_BO(3) ),( 1 - 2*( q_BO(1)^2 + q_BO(2)^2 ) )  ) ;
              asin( 2*(q_BO(4)*q_BO(2)+q_BO(3)*q_BO(1)) );
             atan2( 2*( q_BO(4)*q_BO(3)-q_BO(1)*q_BO(2) ),( 1 - 2*( q_BO(2)^2 + q_BO(3)^2 ) )  ) ];
         
w_BIB = x(5:7);
w_OIO = [0; -s_W_SAT; 0];

q0 = q_BO(4); q1 = q_BO(1); q2 = q_BO(2); q3 = q_BO(3);

TBO = [ q0^2 + q1^2 - q2^2 - q3^2,         2*q0*q3 + 2*q1*q2,         2*q1*q3 - 2*q0*q2;
           2*q1*q2 - 2*q0*q3, q0^2 - q1^2 + q2^2 - q3^2,         2*q0*q1 + 2*q2*q3;
           2*q0*q2 + 2*q1*q3,         2*q2*q3 - 2*q0*q1, q0^2 - q1^2 - q2^2 + q3^2];
       
w_OIB = TBO*w_OIO;
w_BOB = w_BIB - w_OIB;

modw = sqrt(dot(w_BOB,w_BOB));

== matlab function SGP /Subsystem/Embedded MATLAB Function2 ==
  data: t0 parameter double; dn0 parameter double; ddn0 parameter double; Bstar parameter double; i0 parameter double; Ohm0 parameter double; e0 parameter double; w0 parameter double; M0 parameter double; n0 parameter double; revNo parameter double; dT input double; R output double; dR output double
function [R, dR] = sgp(t0,dn0,ddn0,Bstar,i0,Ohm0,e0,w0,M0,n0,revNo,dT)
%This code is a matlab implementation of the SGP Fortran code in the
% Startrack report #3.
%
% The matlab code was derived mainly by porting and editing the
% FORTRAN routines in NORAD’s Spacetrack report #3.
% According to a statement in that report, the document is free
% of copyrights and open to unlimited public distribution.
%
% This matlab code is distributed under the same conditions
%
%
% Created 15/10-2001 by
% Klaus Krogsgaard & Torsten Lorentzen
% - - - - - - - - - - - - - - - - - - - - - - - - -
%
% SGP model for predicting orbit position.
%

% - - - - - - - - - - - - - - - - - - - - - - - - -
% Constants given by the modified NORAD TLE (all at epoch)
% - - - - - - - - - - - - - - - - - - - - - - - - -


% t0 = modTLE(1);
% dn0 = modTLE(2); % first time derivative of the mean motion
% ddn0 = modTLE(3); % second time derivative of mean motion
% Bstar = modTLE(4); % Drag parameter
% i0 = modTLE(5); % inclination
% Ohm0 = modTLE(6); % right ascension of the ascending node
% e0 = modTLE(7); % eccentricity
% w0 = modTLE(8); % argument of perigee
% M0 = modTLE(9); % mean anormaly
% n0 = modTLE(10); % mean motion
% revNo = modTLE(11); % Number of revolutions before epoch
% - - - - - - - - - - - - - - - - - - - - - - - - -
% Other constants
% - - - - - - - - - - - - - - - - - - - - - - - - -
GM = 398603 * 10^9;
er = 6378.135;
ke = 0.0743669161; %converted to er/min ^3/2
% aE = 6378160; % equatorial radius of the Earth
aE = 1;% give result in Earth radii
min_per_day = 1440;
sec_per_day = 86400;
km_per_er = er;
J2 = 5.413080*10^-4 * 2; % second gravitational zonal harmonic of the Earth
J3 = -0.253881*10^-5; % third gravitational zonal harmonic of the Earth
J4 = -0.62098875*10^-6 * 8/3; % fourth gravitational zonal harmonic of the Earth
% - - - - - - - - - - - - - - - - - - - - - - - - -
% Local constants
% - - - - - - - - - - - - - - - - - - - - - - - - -
a1 = (ke/n0)^(2/3);
delta1 = 3/4 * J2 * (aE/a1)^2 * (3*((cos(i0))^2)-1)/((1-e0^2)^(3/2));
a0 = a1 * (1 - 1/3*delta1 - delta1^2 - 134/81*delta1^3);
p0 = a0 * (1 - e0^2);
q0 = a0 * (1-e0);
L0 = M0 + w0 + Ohm0;
dOhm = - (3/2) * J2 * (aE/p0)^2 * n0 * cos(i0);
dw = (3/4) * J2 * (aE/p0)^2 * n0 * (5*(cos(i0))^2-1);
% - - - - - - - - - - - - - - - - - - - - - - - - -
% Secular effects of drag and gravitation
% - - - - - - - - - - - - - - - - - - - - - - - - -
a = a0 * ( n0 ./ (n0 + 2*(dn0/2)*(dT) + 3*(ddn0/6)*dT.^2)).^(2/3); % vector
e = zeros(1,length(dT)); % vector
for i=1:length(a)
if ( a(i)>q0 )
e(i) = 1 - q0/a(i);
else
e(i) = 10^-6;
end;
end;
p = a .* (1-e.^2); % vector
OhmS0 = Ohm0 + dOhm * dT; % vector
wS0 = w0 + dw * (dT); % vector
Ls = mod(L0 + (n0 + dw + dOhm)*(dT) + dn0/2 * (dT).^2 + ddn0/6 * (dT).^3,2*pi); % vector
% - - - - - - - - - - - - - - - - - - - - - - - - -
% Long period periodic effects
% - - - - - - - - - - - - - - - - - - - - - - - - -
axNSL = e .* cos(wS0); % vector
ayNSL = e .* sin(wS0) - 1/2 * J3/J2 * aE./p * sin(i0); % vector
L = mod(Ls - 1/4 * J3/J2 * aE./p .* axNSL * sin(i0) * (3+5*cos(i0))/(1+cos(i0)),2*pi); % vector
% - - - - - - - - - - - - - - - - - - - - - - - - -
% Iteration
% - - - - - - - - - - - - - - - - - - - - - - - - -
tol = 10^-8;
U = mod(L - OhmS0,2*pi); % vector
Ew1 = U; % vector
Ew2 = Ew1; % vector
dEw = (U - ayNSL.*cos(Ew1) + axNSL.*sin(Ew1) - Ew1) ./ (-ayNSL.*sin(Ew1) - axNSL.*cos(Ew1) + 1); % vector
for i=1:length(dEw)
if abs(dEw(i)) > 1
Ew2(i) = Ew1(i) + sign(dEw(i)); %vector
else
Ew2(i) = Ew1(i) + dEw(i);
end;
end;
for i=1:length(Ew1)
while abs(dEw(i))>tol
Ew1(i) = Ew2(i);
dEw(i) = (U(i) - ayNSL(i).*cos(Ew1(i)) + axNSL(i).*sin(Ew1(i)) - Ew1(i)) ./ ...
(-ayNSL(i).*sin(Ew1(i)) - axNSL(i).*cos(Ew1(i)) + 1);
if abs(dEw(i)) > 1
Ew2(i) = Ew1(i) + sign(dEw(i)); %vector
else
Ew2(i) = Ew1(i) + dEw(i);
end;
end;
end;
ecosE = axNSL.*cos(Ew2) + ayNSL.*sin(Ew2); % vector
esinE = axNSL.*sin(Ew2) - ayNSL.*cos(Ew2); % vector
SQeL = axNSL.^2 + ayNSL.^2; % vector
pL = a.*(1 - SQeL); % vector
r = a.*(1 - ecosE); % vector
dr = ke * sqrt(a)./r .* esinE; % vector
rdv = ke * sqrt(pL)./r; % vector
sinu = a./r .* (sin(Ew2) - ayNSL - axNSL.*esinE./(1+sqrt(1-SQeL))); % vector
cosu = a./r .* (cos(Ew2) - axNSL + ayNSL.*esinE./(1+sqrt(1-SQeL))); % vectro
u = mod(atan2( sinu,cosu ),2*pi); % vector
% - - - - - - - - - - - - - - - - - - - - - - - - -
% Short term perturbations
% - - - - - - - - - - - - - - - - - - - - - - - - -
rk = r + 1/4 * J2 * aE^2./pL * (sin(i0))^2 .* cos(2*u); % vector
uk = u - 1/8 * J2 * (aE./pL).^2 * (7 * (cos(i0))^2 - 1) .* sin(2*u); % vector
Ohmk = OhmS0 + 3/4 * J2 * (aE./pL).^2 * cos(i0) .* sin(2*u); % vector
ik = i0 + 3/4 * J2 * (aE./pL).^2 * sin(i0) * cos(i0) .* cos(2*u); % vector
% - - - - - - - - - - - - - - - - - - - - - - - - -
% Unit orientation vectors
% - - - - - - - - - - - - - - - - - - - - - - - - -
R = zeros(length(uk),3); % vector
dR = zeros(length(uk),3); % vector
for i=1:length(uk)
    M_vec = [ -sin(Ohmk(i))*cos(ik(i)) cos(Ohmk(i))*cos(ik(i)) sin(ik(i)) ]; % vector
N_vec = [ cos(Ohmk(i)) sin(Ohmk(i)) 0 ]; % vector
U_vec = M_vec * sin(uk(i)) + N_vec * cos(uk(i)); % vector
V_vec = M_vec * cos(uk(i)) - N_vec * sin(uk(i)); % vector
% - - - - - - - - - - - - - - - - - - - - - - - - -
% Position and velocity
% - - - - - - - - - - - - - - - - - - - - - - - - -
R(i,:) = rk(i) * U_vec; % vector
dR(i,:) = dr(i) * U_vec + rdv(i) * V_vec; % vector
end;
% - - - - - - - - - - - - - - - - - - - - - - - - -
% Transforming position to Cartesian coordinates in kilometers and velocity to kilometers/sec
% - - - - - - - - - - - - - - - - - - - - - - - - -
R = R * km_per_er /aE;
R = R * 1000; % km to m
dR = dR * km_per_er / aE * min_per_day / sec_per_day;
dR = dR * 1000; % km/s to m/s
